simulink subsystem "PowertrainMatlab"  (R2025b)
settings: Solver=VariableStepAuto  StartTime=0.0  StopTime=10.0  RelTol=1e-3
settings Model: Creator=bigch  LastModifiedBy=jessi

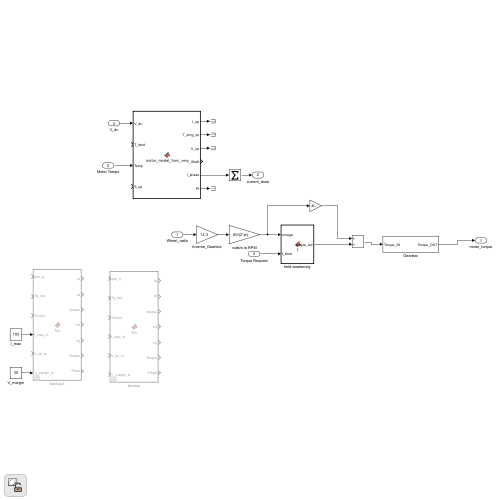
[thumbnail: Simulink's stored preview of the top-level diagram]
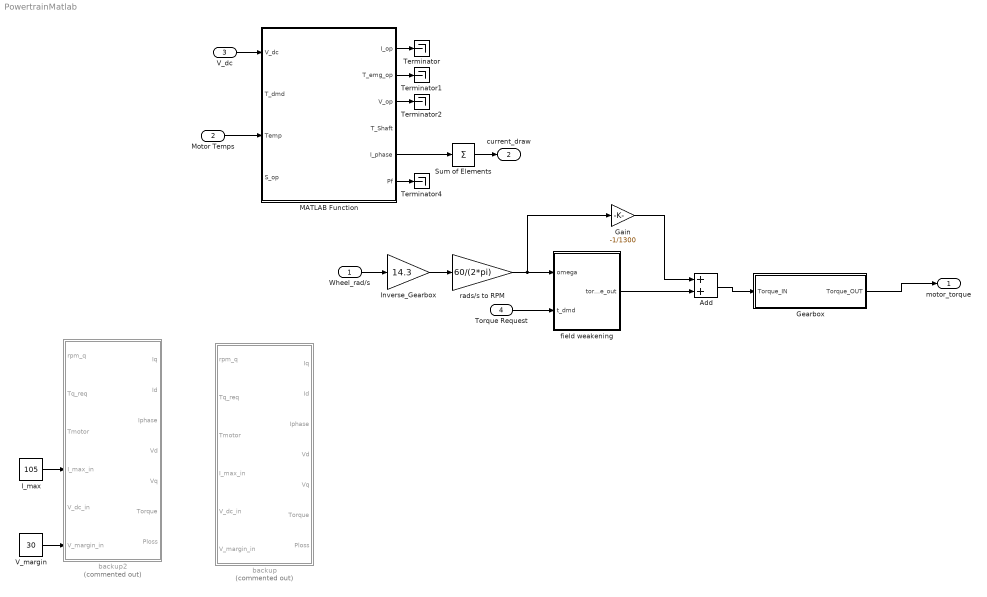
== system PowertrainMatlab ==
  Wheel_rad/s : Inport  Unit=rpm  PortDimensions=4
  Motor Temps : Inport  Port=2  Unit=°C  PortDimensions=4
  V_dc : Inport  Port=3  Unit=V  PortDimensions=1
  Torque Request : Inport  Port=4  Unit=N*m  PortDimensions=4
  Add : Sum
  Gain : Gain  Gain=-1/1300
  Gearbox : Subsystem
  I_max : Constant  Value=105
  Inverse_Gearbox : Gain  Gain=14.3
  MATLAB Function : MATLAB Function  TreatAsAtomicUnit=on
  Sum of Elements : Sum  Inputs=+
  Terminator{,1..2,4} (4 alike) : Terminator
  V_margin : Constant  Value=30
  backup : MATLAB Function  Commented=on  TreatAsAtomicUnit=on
  backup2 : MATLAB Function  Commented=on  TreatAsAtomicUnit=on
  field weakening : MATLAB Function  TreatAsAtomicUnit=on
  rads/s to RPM : Gain  Gain=60/(2*pi)
  motor_torque : Outport  Unit=N*m  PortDimensions=4
  current_draw : Outport  Port=2  Unit=A  PortDimensions=1
  wires:
  MATLAB Function/6(Pf) -> Terminator4/1
  MATLAB Function/3(V_op) -> Terminator2/1
  MATLAB Function/2(T_emg_op) -> Terminator1/1
  MATLAB Function/1(I_op) -> Terminator/1
  V_dc/1 -> MATLAB Function/1(V_dc)
  V_margin/1 -> backup2/6(V_margin_in)
  Motor Temps/1 -> MATLAB Function/3(Temp)
  I_max/1 -> backup2/4(I_max_in)
  Sum of Elements/1 -> current_draw/1
  MATLAB Function/5(I_phase) -> Sum of Elements/1
  Torque Request/1 -> field weakening/2(t_dmd)
  Gearbox/1(Torque_OUT) -> motor_torque/1
  field weakening/1(torque_out) -> Add/2
  Add/1 -> Gearbox/1(Torque_IN)
  rads/s to RPM/1 -> field weakening/1(omega), Gain/1
  Gain/1 -> Add/1
  Wheel_rad/s/1 -> Inverse_Gearbox/1
  Inverse_Gearbox/1 -> rads/s to RPM/1

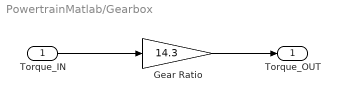
== system PowertrainMatlab/Gearbox ==
  Torque_IN : Inport
  Gear Ratio : Gain  Gain=14.3
  Torque_OUT : Outport
  wires:
  Torque_IN/1 -> Gear Ratio/1
  Gear Ratio/1 -> Torque_OUT/1

== matlab function PowertrainMatlab/MATLAB Function ==
  data: V_dc input; T_dmd input; Temp input; S_op input; I_op output; T_emg_op output; V_op output; T_Shaft output; I_phase output; Pf output
function [I_op, T_emg_op, V_op, T_Shaft, I_phase, Pf] = motor_model_func_vec(V_dc, T_dmd, Temp, S_op)
    nn = size(T_dmd);
    n = nn(1);
    I_op = zeros(n, 1);
    T_emg_op = zeros(n, 1);
    V_op = zeros(n, 1);
    T_Shaft = zeros(n, 1);
    I_phase = zeros(n, 1);
    Pf = zeros(n);
    for i = 1:n
        [I_op(i), T_emg_op(i), V_op(i), T_Shaft(i), I_phase(i), Pf(i)] = motor_model_func(V_dc,T_dmd(i), Temp(i), S_op(i));
    end
end

function [I_op, T_emg_op, V_op, T_Shaft, I_phase, Pf] = motor_model_func(V_dc,T_dmd, Temp, S_op)
% Inputs:
%   V_dc  - DC bus / peak-phase voltage limit (V)
%   T_dmd - requested electromagnetic torque (Nm)
%   Temp  - requested motor temperature (degC) (use 80-120 ideally)
%   S_op  - operating speed (rpm) at which to find operating point
%
% Output (struct res)
%   res.I_op       - approximated phase current (A) corresponding to column
%   res.T_emg_op   - Electromagnetic torque value found (Nm)
%   res.V_op       - phase-peak voltage found (same units as Voltage_Phase_Peak)
%   res.T_Shaft    - shaft torque (usable torque) (Nm)
%   res.I_phase    - stator phase current (ARMS)
%   res.Mech_loss  - mechanical loss (W)
%   res.Pf         - power factor
%
% Notes:
%   - Implementation chooses two temp files T1/T2 surrounding Temp, 
%     interpolates across speed to evaluate T and V at S_op, sweeps currents 
%     low->high to find exact or interpolated torque match, then interpolates
%     other maps between T1/T2 to produce final outputs.m,

    [data80, data100, data120] = coder.const(@load_data);
    rows = 201;
    cols = 21;
    
    if Temp <= 80
        t1 = data80;
        t2 = data80;
        fracT = 0;
    elseif 80 < Temp && Temp <= 100
        t1 = data80;
        t2 = data100;
        fracT = (Temp - 80)/(100-80);
    elseif 100 <= Temp && Temp < 120
        t1 = data100;
        t2 = data120;
        fracT = (Temp-100)/(120-100);
    else
        t1 = data120;
        t2 = data120;
        fracT = 1;
    end

    % round S_op to nearest increment of 20000/rows
    speed_inc = 20000/(rows - 1);
    S_idx = abs(S_op / speed_inc) + 1;
    current_inc = 105/(cols - 1);
    
    % find current limit from voltage
    V = bilinear_interpolation(t1.Voltage_Phase_Peak, t2.Voltage_Phase_Peak, S_idx, fracT);
    V_find = find(diff(V > V_dc) == 1, 1); % find lmao
    if isempty(V_find)
        % figure out if you are too low or too high
        if V_dc < V(1)
            V_cur_lim_idx = 1;
        else
            V_cur_lim_idx = cols;
        end
    else
        % note that tq_find+1 as tq_find in [1,n-1] (as difference array
        % removes an element at the end)
        V_cur_lim_idx = V_find + (V_dc - V(V_find))/(V(V_find + 1) - V(V_find));
    end

    % find current required for torque
    Tq = bilinear_interpolation(t1.Electromagnetic_Torque, t2.Electromagnetic_Torque, S_idx, fracT);
    Tq_find = find(diff(Tq > T_dmd) == 1, 1); % find lmao
    if isempty(Tq_find)
        % figure out if you are too low or too high
        if T_dmd < Tq(1)
            Tq_cur_lim_idx= 1;
        else
            Tq_cur_lim_idx = cols;
        end
    else
        % note that tq_find+1 as tq_find in [1,n-1] (as difference array
        % removes an element at the end)
        Tq_cur_lim_idx = Tq_find + (T_dmd - Tq(Tq_find))/(Tq(Tq_find + 1) - Tq(Tq_find));
    end
    
    % find the current draw
    %fprintf("Voltage Current Limit: %fA, Torque Current Limit: %fA\n", (V_cur_lim_idx - 1) * current_inc, (Tq_cur_lim_idx - 1) * current_inc);
    I_idx = min(Tq_cur_lim_idx, V_cur_lim_idx);

    %fprintf("Speed Interp: %f Current Interp: %f Temperature Interp: %f\n", S_idx, I_idx, fracT);
    %fprintf("Speed: %fRPM Current: %fA\n", S_idx * speed_inc, (I_idx-1) * current_inc);

    I_op = (I_idx-1) * current_inc; % stupid ahh 1 indexing
    T_emg_op = trilinear_query(t1.Electromagnetic_Torque, t2.Electromagnetic_Torque, S_idx, I_idx, fracT);
    V_op = trilinear_query(t1.Voltage_Phase_Peak, t2.Voltage_Phase_Peak, S_idx, I_idx, fracT);
    T_Shaft = trilinear_query(t1.Shaft_Torque, t2.Shaft_Torque, S_idx, I_idx, fracT);
    I_phase = trilinear_query(t1.Stator_Current_Phase_RMS, t2.Stator_Current_Phase_RMS, S_idx, I_idx, fracT);
    Pf = trilinear_query(t1.Power_Factor, t2.Power_Factor, S_idx, I_idx, fracT);
end

function [data80, data100, data120] = load_data()
    data80 = coder.load("A2370DD_T80C.mat");
    data100 = coder.load("A2370DD_T100C.mat");
    data120 = coder.load("A2370DD_T120C.mat");
end

% quicky bilinear interpolation
function m = bilinear_interpolation(mat_t1, mat_t2, S_idx, fracT)
    % S_idx is the decimal index of speed. The integer part represents the
    % lower bound speed and the fraction part represents the amount to
    % interpolate
    % fracT represents the weighting to give between mat_t1 and mat_t2
    S_idx_lb = fix(S_idx);
    fracS = S_idx - S_idx_lb;
    S_idx_ub = S_idx_lb + 1; % this should be safe as is fracS = 0, then it should short circuit the multiplication calculation

    % we choose to interpolate on speed first because it reduces the
    % dimension of the array
    m_at_Sop_1 = (1-fracS)*mat_t1(S_idx_lb, :) + fracS*mat_t1(S_idx_ub, :);
    m_at_Sop_2 = (1-fracS)*mat_t2(S_idx_lb, :) + fracS*mat_t2(S_idx_ub, :);
    % then interpolate on motor temperature
    m = (1-fracT)*m_at_Sop_1 + fracT*m_at_Sop_2;
end

function val = trilinear_query(mat_t1, mat_t2, S_idx, I_idx, fracT)
    m = bilinear_interpolation(mat_t1, mat_t2, S_idx, fracT);
    I_idx_lb = fix(I_idx);
    fracI = I_idx - I_idx_lb;
    I_idx_ub = I_idx_lb + 1;
    val = (1 - fracI)*m(I_idx_lb) + fracI*m(I_idx_ub);
end

== matlab function PowertrainMatlab/backup2 ==
  settings: updateMethod=CONTINUOUS
  data: rpm_q input; Iq output; Tq_req input; Tmotor input; I_max_in input; V_dc_in input; V_margin_in input; Id output; Iphase output; Vd output; Vq output; Torque output; Ploss output
function [Iq, Id, Iphase, Vd, Vq, Torque, Ploss] =  fcn(rpm_q, Tq_req, Tmotor, I_max_in, V_dc_in, V_margin_in)
    [maps80, maps120] = coder.const(@test);
    limits = struct();
    limits.I_max = I_max_in;
    limits.V_margin = V_margin_in;
    limits.V_dc = V_dc_in; 
    
    % The alpha interpolation calculation
    alpha = max(min((Tmotor-80)/(120-80), 1), 0);
    
    % Interpolated values (Now using the persistent maps)
    Iq = (1-alpha)*maps80.Iq_RMS(rpm_q,Tq_req)   + alpha*maps120.Iq_RMS(rpm_q,Tq_req);
    Id = (1-alpha)*maps80.Id_RMS(rpm_q,Tq_req)   + alpha*maps120.Id_RMS(rpm_q,Tq_req);
    Iphase = (1-alpha)*maps80.Stator_Current_Phase_RMS(rpm_q,Tq_req) ...
                    + alpha*maps120.Stator_Current_Phase_RMS(rpm_q,Tq_req);
    Vd = (1-alpha)*maps80.Vd_RMS(rpm_q,Tq_req)   + alpha*maps120.Vd_RMS(rpm_q,Tq_req);
    Vq = (1-alpha)*maps80.Vq_RMS(rpm_q,Tq_req)   + alpha*maps120.Vq_RMS(rpm_q,Tq_req);
    Torque = (1-alpha)*maps80.Shaft_Torque(rpm_q,Tq_req) + alpha*maps120.Shaft_Torque(rpm_q,Tq_req);
    Ploss  = (1-alpha)*maps80.Total_Loss(rpm_q,Tq_req)   + alpha*maps120.Total_Loss(rpm_q,Tq_req);
    
    % Current limit (Now using persistent limits)
    if Iphase > limits.I_max
        scale   = limits.I_max / Iphase;
        Iq  = Iq*scale; 
        Id  = Id*scale;
        Torque  = Torque*scale;
        Iphase  = limits.I_max;
    end
    
    % Voltage limit (Now using persistent limits)
    V_lim = (limits.V_dc - limits.V_margin)/sqrt(3);
    V_req = sqrt(Vd^2 + Vq^2);
    if V_req > V_lim
        Torque = Torque * (V_lim/V_req);
    end
end

function [maps80, maps120] = test()
    % Load MAT files
    data80  = coder.load('A2370DD_T80C.mat');
    data120 = coder.load('A2370DD_T120C.mat');
    % Axes setup
    rpm_vec = data80.Speed(:,1);          
    T_vec   = data80.Shaft_Torque(1,:);   
    
    % Build gridded interpolnts
    fields = {'Shaft_Torque','Id_RMS','Iq_RMS','Stator_Current_Phase_RMS',...
              'Vd_RMS','Vq_RMS','Total_Loss','Stator_Copper_Loss',...
              'Iron_Loss','Magnet_Loss','Mechanical_Loss'};
    maps80 = struct(); 
    maps120 = struct();
    for i = 1:length(fields)
        f = fields{i};
        maps80.(f)  = griddedInterpolant({rpm_vec, T_vec}, data80.(f),  'linear','nearest');
        maps120.(f) = griddedInterpolant({rpm_vec, T_vec}, data120.(f), 'linear','nearest');
    end
end

== matlab function PowertrainMatlab/field weakening ==
  data: omega input; torque_out output; t_dmd input
function torque_out = f(omega, t_dmd)
    torque_out = min(max(0, -0.0034 * omega + 68.6), t_dmd);
end

== matlab function PowertrainMatlab/backup ==
  settings: updateMethod=CONTINUOUS
  data: rpm_q input; Iq output; Tq_req input; Tmotor input; I_max_in input; V_dc_in input; V_margin_in input; Id output; Iphase output; Vd output; Vq output; Torque output; Ploss output
function [Iq, Id, Iphase, Vd, Vq, Torque, Ploss]= fcn(rpm_q,Tq_req, Tmotor, I_max_in, V_dc_in, V_margin_in)
   
    persistent maps80 maps120 limits I_max V_margin
  
    if isempty(maps80)
        
        I_max = I_max_in;
        V_margin = V_margin_in;
        
        % Load MAT files
        data80  = coder.load('A2370DD_T80C.mat');
        data120 = coder.load('A2370DD_T120C.mat');
       
        % Axes setup
        rpm_vec = data80.Speed(:,1);          
        T_vec   = data80.Shaft_Torque(1,:);   
        
        % Build gridded interpolnts
        fields = {'Shaft_Torque','Id_RMS','Iq_RMS','Stator_Current_Phase_RMS',...
                  'Vd_RMS','Vq_RMS','Total_Loss','Stator_Copper_Loss',...
                  'Iron_Loss','Magnet_Loss','Mechanical_Loss'};
        maps80 = struct(); 
        maps120 = struct();
        for i = 1:length(fields)
            f = fields{i};
            maps80.(f)  = griddedInterpolant({rpm_vec, T_vec}, data80.(f),  'linear','nearest');
            maps120.(f) = griddedInterpolant({rpm_vec, T_vec}, data120.(f), 'linear','nearest');
        end
        
        limits = struct();
        limits.I_max = I_max;
        limits.V_margin = V_margin;
        
        
    end

    limits.V_dc = V_dc_in; 
    
    % --- RUNTIME CODE (The only part that runs every step) ---
    
    % The alpha interpolation calculation
    alpha = max(min((Tmotor-80)/(120-80), 1), 0);
    
    % Interpolated values (Now using the persistent maps)
    Iq = (1-alpha)*maps80.Iq_RMS(rpm_q,Tq_req)   + alpha*maps120.Iq_RMS(rpm_q,Tq_req);
    Id = (1-alpha)*maps80.Id_RMS(rpm_q,Tq_req)   + alpha*maps120.Id_RMS(rpm_q,Tq_req);
    Iphase = (1-alpha)*maps80.Stator_Current_Phase_RMS(rpm_q,Tq_req) ...
                    + alpha*maps120.Stator_Current_Phase_RMS(rpm_q,Tq_req);
    Vd = (1-alpha)*maps80.Vd_RMS(rpm_q,Tq_req)   + alpha*maps120.Vd_RMS(rpm_q,Tq_req);
    Vq = (1-alpha)*maps80.Vq_RMS(rpm_q,Tq_req)   + alpha*maps120.Vq_RMS(rpm_q,Tq_req);
    Torque = (1-alpha)*maps80.Shaft_Torque(rpm_q,Tq_req) + alpha*maps120.Shaft_Torque(rpm_q,Tq_req);
    Ploss  = (1-alpha)*maps80.Total_Loss(rpm_q,Tq_req)   + alpha*maps120.Total_Loss(rpm_q,Tq_req);
    
    % Current limit (Now using persistent limits)
    if Iphase > limits.I_max
        scale   = limits.I_max / Iphase;
        Iq  = Iq*scale; 
        Id  = Id*scale;
        Torque  = Torque*scale;
        Iphase  = limits.I_max;
    end
    
    % Voltage limit (Now using persistent limits)
    V_lim = (limits.V_dc - limits.V_margin)/sqrt(3);
    V_req = sqrt(Vd^2 + Vq^2);
    if V_req > V_lim
        Torque = Torque * (V_lim/V_req);
    end
   

end
